simulink model "test_passabasso"  (R2023a)
settings: Solver=VariableStepAuto  StartTime=0.0  StopTime=50  RelTol=1e-3
undefined symbols (not defined in the file or in its folder): passa_basso
libraries: dspsrcs4 x1
settings Model: Creator=peter  LastModifiedBy=edoar
settings OptimizationCC: ReuseModelBlockBuffer=off

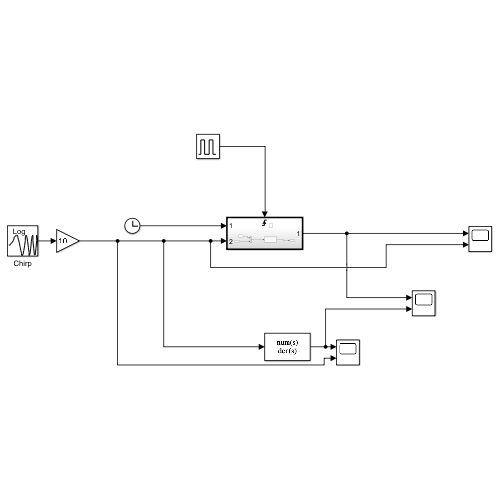
[thumbnail: Simulink's stored preview of the top-level diagram]
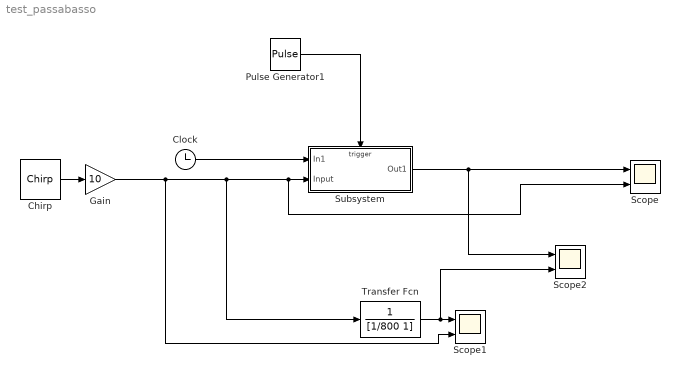
== system test_passabasso ==
  Chirp : dspsrcs4/Chirp  sweep=Logarithmic  mode=Unidirectional  f0=0.1  f1=20000  t1=50  Tsweep=50  phase=0  Ts=0.001  spf=1  datatype=Double  OutputFrames=off
  Clock : Clock
      settings: Decimation=100000
  Gain : Gain  Gain=10
  Pulse Generator1 : DiscretePulseGenerator  PulseType=Time based  Period=0.001  PulseWidth=50
  Scope : Scope  NumInputPorts=2
  Scope1 : Scope  NumInputPorts=2
  Scope2 : Scope  NumInputPorts=2
  Subsystem : Subsystem
  Transfer Fcn : TransferFcn  Denominator=[1/800 1]
  wires:
  Pulse Generator1/1 -> Subsystem/Trigger
  Clock/1 -> Subsystem/1(In1)
  Subsystem/1(Out1) -> Scope2/1, Scope/1
  Transfer Fcn/1 -> Scope2/2, Scope1/1
  Chirp/1 -> Gain/1
  Gain/1 -> Scope1/2, Transfer Fcn/1, Scope/2, Subsystem/2(Input)

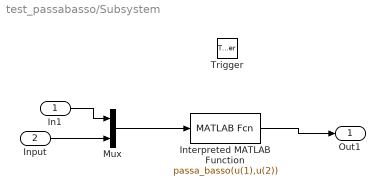
== system test_passabasso/Subsystem ==
  In1 : Inport
  Input : Inport  Port=2
  Trigger : TriggerPort  VariantControl=(inherit)  PortDimensions=1
  Interpreted MATLAB Function : MATLABFcn  MATLABFcn=passa_basso(u(1),u(2))
  Mux : Mux  Inputs=2
  Out1 : Outport
  wires:
  Mux/1 -> Interpreted MATLAB Function/1
  In1/1 -> Mux/1
  Interpreted MATLAB Function/1 -> Out1/1
  Input/1 -> Mux/2
